simulink model "Belousov_Zhabotinsky"  (R2014b)
settings: Solver=ode45  StartTime=0.0  StopTime=10.0  RelTol=1e-3
values from neighbouring files (symbols this model uses):
  d = 4 * 1e-3    (= 0.004)    [Run_Belousov_Zhabotinsky.m]    (also in Run_HindmarshRose.m = 5; Run_Qi_4D.m = 0.6; Run_Roessler_4D.m = 0.05)
  f = 1.05    [Run_Belousov_Zhabotinsky.m]
  q = 8 * 1e-4    (= 0.0008)    [Run_Belousov_Zhabotinsky.m]
undefined symbols (not defined in the file or in its folder): param
settings Model: Creator=Arek  LastModifiedBy=Arek

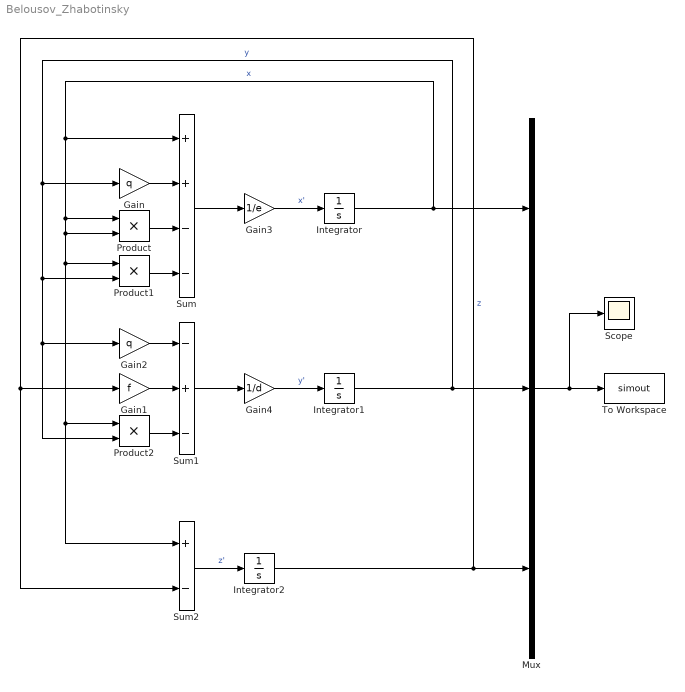
== system Belousov_Zhabotinsky ==
  Gain : Gain  Gain=q
  Gain1 : Gain  Gain=f
  Gain2 : Gain  Gain=q
  Gain3 : Gain  Gain=1/e
  Gain4 : Gain  Gain=1/d
  Integrator : Integrator  InitialCondition=param.ic(1)
  Integrator1 : Integrator  InitialCondition=param.ic(2)
  Integrator2 : Integrator  InitialCondition=param.ic(3)
  Mux : Mux  Inputs=3
  Product : Product
  Product1 : Product
  Product2 : Product
  Scope : Scope
      settings: ShowLegends=on
  Sum : Sum  Inputs=++--
  Sum1 : Sum  Inputs=-+-
  Sum2 : Sum  Inputs=+-
  To Workspace : ToWorkspace  VariableName=simout  SaveFormat=Timeseries  SampleTime=-1
  wires:
  Integrator/1 -> Product/1, Product/2, Product1/1, Sum2/1, Product2/1, Sum/1, Mux/1  "x"
  Gain4/1 -> Integrator1/1  "y'"
  Integrator1/1 -> Product1/2, Gain2/1, Product2/2, Gain/1, Mux/2  "y"
  Sum2/1 -> Integrator2/1  "z'"
  Integrator2/1 -> Sum2/2, Gain1/1, Mux/3  "z"
  Mux/1 -> Scope/1, To Workspace/1
  Gain3/1 -> Integrator/1  "x'"
  Gain/1 -> Sum/2
  Product1/1 -> Sum/4
  Product/1 -> Sum/3
  Gain2/1 -> Sum1/1
  Product2/1 -> Sum1/3
  Gain1/1 -> Sum1/2
  Sum/1 -> Gain3/1
  Sum1/1 -> Gain4/1
